simulink model "noisy_minorder"  (R2025b)
settings: Solver=VariableStepAuto  StartTime=0.0  StopTime=400  RelTol=1e-3
values from neighbouring files (symbols this model uses):
  A = [0 -0.0122335357927 0 0.04653303839 1 0 0 0 0 -2.91800139921 0 37.7525456689 ... (16 elements, 4x4)]    [matlab.mat]
  B = [0 -0.714154574773 0 -0.000498818992568]    [matlab.mat]
  C = [1 0 0 0 0 1 0 0 0 0 1 0 ... (16 elements, 4x4)]    [matlab.mat]
  K_lqr = [-1231.62178055 75.4404321566 -1810304.48785 -294623.729953]    [matlab.mat]
undefined symbols (not defined in the file or in its folder): a, A_obs, b, B_obs, C_obs, D_obs, F_obs
libraries: simulink x1
settings Model: Creator=shree  LastModifiedBy=shree

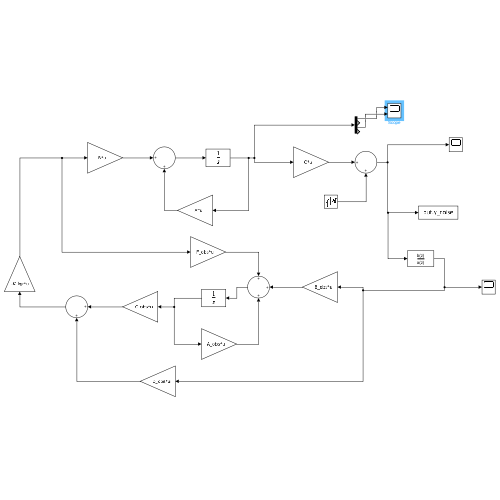
[thumbnail: Simulink's stored preview of the top-level diagram]
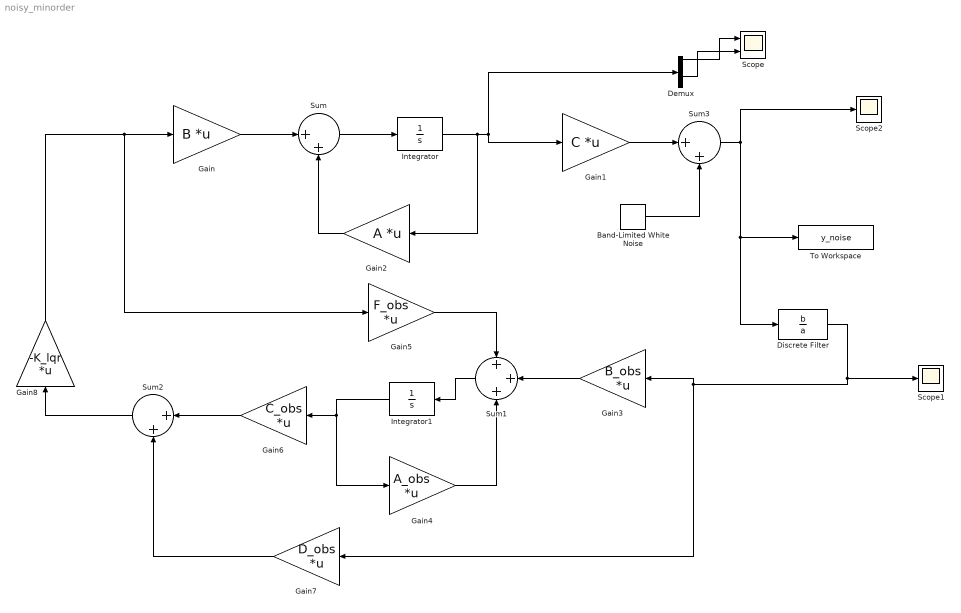
== system noisy_minorder ==
  Band-Limited White Noise : simulink/Sources/Band-Limited White Noise  Cov=[0.00000000001]  Ts=0.00001  seed=[23341]
  Demux : Demux
  Discrete Filter : DiscreteFilter  Numerator=b  Denominator=a
  Gain : Gain  Gain=B  Multiplication=Matrix(K*u)
  Gain1 : Gain  Gain=C  Multiplication=Matrix(K*u)
  Gain2 : Gain  Gain=A  Multiplication=Matrix(K*u)
  Gain3 : Gain  Gain=B_obs  Multiplication=Matrix(K*u)
  Gain4 : Gain  Gain=A_obs  Multiplication=Matrix(K*u)
  Gain5 : Gain  Gain=F_obs  Multiplication=Matrix(K*u)
  Gain6 : Gain  Gain=C_obs  Multiplication=Matrix(K*u)
  Gain7 : Gain  Gain=D_obs  Multiplication=Matrix(K*u)
  Gain8 : Gain  Gain=-K_lqr  Multiplication=Matrix(K*u)
  Integrator : Integrator  InitialCondition=[0.01,0,0.087266,0]
  Integrator1 : Integrator  InitialCondition=[-0.02, 0 ,0]
  Scope : Scope  NumInputPorts=2
      settings: SampleTime=1e-4  ActiveDisplayYMinimum=-0.087463773174391066  ActiveDisplayYMaximum=0.11361982199558064
  Scope1 : Scope
      settings: SampleTime=1e-4  ActiveDisplayYMinimum=-0.024777238799250922  ActiveDisplayYMaximum=0.10387089901658957
  Scope2 : Scope
      settings: SampleTime=1e-4  ActiveDisplayYMinimum=-0.02560961605305332  ActiveDisplayYMaximum=0.10057178733111791  DataLoggingVariableName=ScopeData2
  Sum : Sum  Inputs=|++
  Sum1 : Sum  Inputs=+++
  Sum2 : Sum  Inputs=|++
  Sum3 : Sum  Inputs=|++
  To Workspace : ToWorkspace  VariableName=y_noise  SaveFormat=Structure With Time  SampleTime=1e-4
  wires:
  Sum1/1 -> Integrator1/1
  Gain6/1 -> Sum2/1
  Sum2/1 -> Gain8/1
  Gain4/1 -> Sum1/3
  Gain8/1 -> Gain5/1, Gain/1
  Gain/1 -> Sum/1
  Integrator/1 -> Gain2/1, Demux/1, Gain1/1
  Gain3/1 -> Sum1/2
  Integrator1/1 -> Gain4/1, Gain6/1
  Gain2/1 -> Sum/2
  Gain5/1 -> Sum1/1
  Gain7/1 -> Sum2/2
  Demux/1 -> Scope/1
  Sum/1 -> Integrator/1
  Gain1/1 -> Sum3/1
  Band-Limited White Noise/1 -> Sum3/2
  Sum3/1 -> Discrete Filter/1, To Workspace/1, Scope2/1
  Discrete Filter/1 -> Gain3/1, Gain7/1, Scope1/1
  Demux/3 -> Scope/2
